simulink model "Salient_Pole_PMSG"  (R2023a)
settings: Solver=VariableStepAuto  StartTime=0.0  StopTime=10.0  RelTol=1e-3
values from neighbouring files (symbols this model uses):
  B = 0.01*Pr/(Wr^2)    (= 0.243170840742)    [SHARKS_PMSG.m]
  J = 0.2564    [SHARKS_PMSG.m]
  lamda_fd = 3*2*k/P    [SHARKS_PMSG.m]
  Lsd = 45.25e-3    (= 0.04525)    [SHARKS_PMSG.m]
  Lsq = 64.88e-3    (= 0.06488)    [SHARKS_PMSG.m]
  P = 24    [SHARKS_PMSG.m]
  Rs = 3.711    [SHARKS_PMSG.m]
libraries: spsabctodq0Lib x1
settings Model: Creator=tariq  LastModifiedBy=tariq

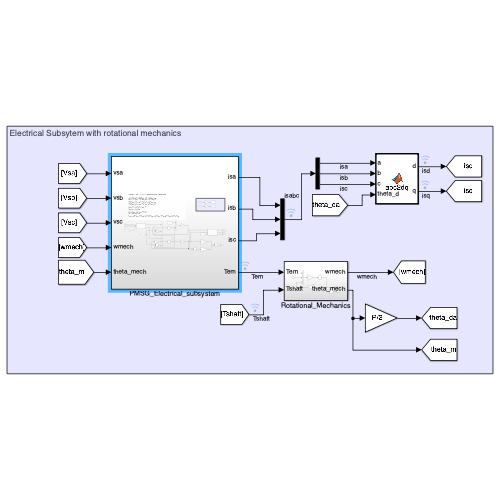
[thumbnail: Simulink's stored preview of the top-level diagram]
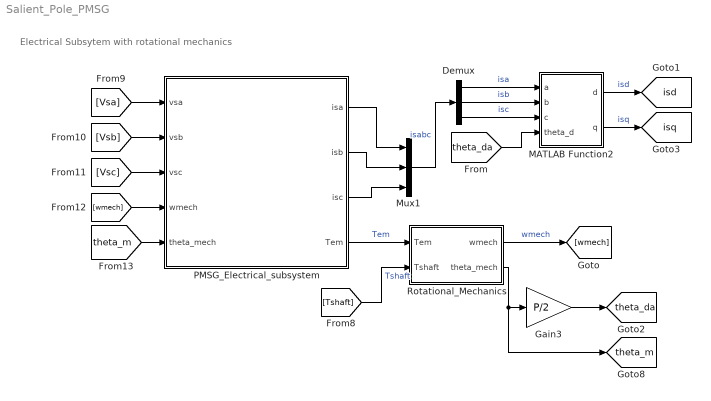
== system Salient_Pole_PMSG ==
  note: Electrical Subsytem with rotational mechanics
  Demux : Demux  Outputs=3
  Gain3 : Gain  Gain=P/2
  MATLAB Function2 : MATLAB Function  TreatAsAtomicUnit=on
  Mux1 : Mux  Inputs=3
  PMSG_Electrical_subsystem : Subsystem
  Rotational_Mechanics : Subsystem
  tag scope: isd=global, isq=global, theta_da=global, theta_m=global
  wires:
  [theta_da] -> MATLAB Function2/4(theta_d)
  Rotational_Mechanics/2(theta_mech) -> [theta_m], Gain3/1
  [Vsc] -> PMSG_Electrical_subsystem/3(vsc)
  Demux/3 -> MATLAB Function2/3(c)  "isc"
  Demux/1 -> MATLAB Function2/1(a)  "isa"
  [theta_m] -> PMSG_Electrical_subsystem/5(theta_mech)
  PMSG_Electrical_subsystem/4(Tem) -> Rotational_Mechanics/1(Tem)  "Tem"
  [Vsa] -> PMSG_Electrical_subsystem/1(vsa)
  [wmech] -> PMSG_Electrical_subsystem/4(wmech)
  MATLAB Function2/2(q) -> [isq]  "isq"
  Mux1/1 -> Demux/1  "isabc"
  [Vsb] -> PMSG_Electrical_subsystem/2(vsb)
  PMSG_Electrical_subsystem/2(isb) -> Mux1/2
  Rotational_Mechanics/1(wmech) -> [wmech]  "wmech"
  Gain3/1 -> [theta_da]
  PMSG_Electrical_subsystem/3(isc) -> Mux1/3
  MATLAB Function2/1(d) -> [isd]  "isd"
  Demux/2 -> MATLAB Function2/2(b)  "isb"
  PMSG_Electrical_subsystem/1(isa) -> Mux1/1
  [Tshaft] -> Rotational_Mechanics/2(Tshaft)  "Tshaft"

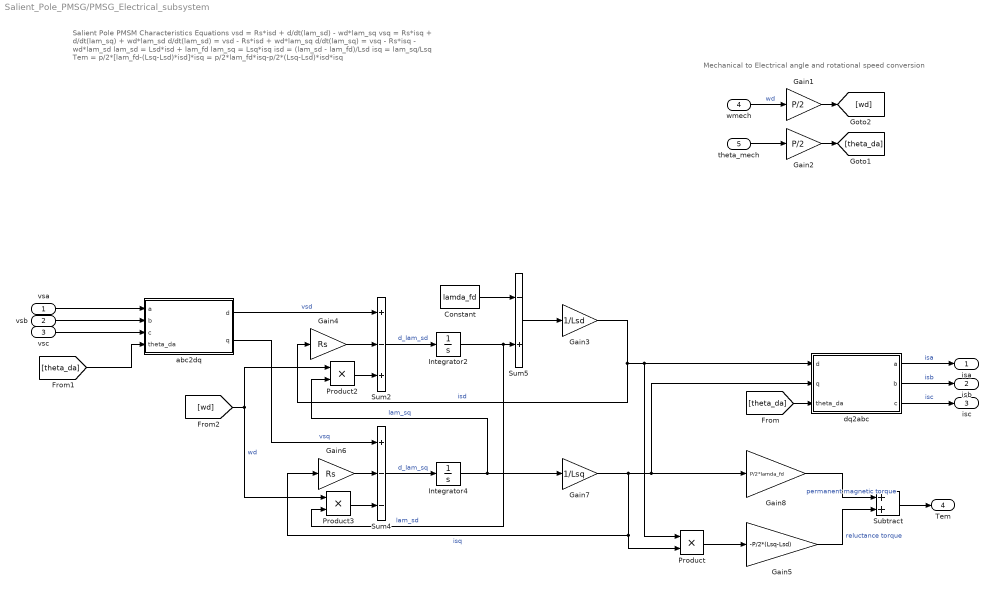
== system Salient_Pole_PMSG/PMSG_Electrical_subsystem ==
  note: Mechanical to Electrical angle and rotational speed conversion
  note: Salient Pole PMSM Characteristics Equations
      |
      | vsd = Rs*isd + d/dt(lam_sd) - wd*lam_sq
      | vsq = Rs*isq + d/dt(lam_sq) + wd*lam_sd
      |
      | d/dt(lam_sd) = vsd - Rs*isd + wd*lam_sq
      | d/dt(lam_sq) = vsq - Rs*isq - wd*lam_sd
      |
      | lam_sd = Lsd*isd + lam_fd
      | lam_sq = Lsq*isq
      |
      | isd = (lam_sd - lam_fd)/Lsd
      | isq = lam_sq/Lsq
      |
      | Tem = p/2*[lam_fd-(Lsq-Lsd)*isd]*isq = p/2*lam_fd*isq-p/2*(Lsq-Lsd)*isd*isq
  vsa : Inport
  vsb : Inport  Port=2
  vsc : Inport  Port=3
  wmech : Inport  Port=4
  theta_mech : Inport  Port=5
  Constant : Constant  Value=lamda_fd
  Gain1 : Gain  Gain=P/2
  Gain2 : Gain  Gain=P/2
  Gain3 : Gain  Gain=1/Lsd
  Gain4 : Gain  Gain=Rs
  Gain5 : Gain  Gain=-P/2*(Lsq-Lsd)
  Gain6 : Gain  Gain=Rs
  Gain7 : Gain  Gain=1/Lsq
  Gain8 : Gain  Gain=P/2*lamda_fd
  Integrator2 : Integrator
  Integrator4 : Integrator
  Product : Product
  Product2 : Product
  Product3 : Product
  Subtract : Sum
  Sum2 : Sum  Inputs=+-+
  Sum4 : Sum  Inputs=+--
  Sum5 : Sum  Inputs=-+
  abc2dq : Subsystem
  dq2abc : Subsystem
  isa : Outport  VectorParamsAs1DForOutWhenUnconnected=off
  isb : Outport  Port=2  VectorParamsAs1DForOutWhenUnconnected=off
  isc : Outport  Port=3  VectorParamsAs1DForOutWhenUnconnected=off
  Tem : Outport  Port=4  VectorParamsAs1DForOutWhenUnconnected=off
  wires:
  vsb/1 -> abc2dq/2(b)
  abc2dq/1(d) -> Sum2/1  "vsd"
  abc2dq/2(q) -> Sum4/1  "vsq"
  [theta_da] -> dq2abc/3(theta_da)
  vsc/1 -> abc2dq/3(c)
  dq2abc/1(a) -> isa/1  "isa"
  dq2abc/2(b) -> isb/1  "isb"
  Gain7/1 -> dq2abc/2(q), Gain8/1, Product/2, Gain6/1  "isq"
  dq2abc/3(c) -> isc/1  "isc"
  vsa/1 -> abc2dq/1(a)
  Gain3/1 -> Product/1, dq2abc/1(d), Gain4/1  "isd"
  Gain4/1 -> Sum2/2
  Product2/1 -> Sum2/3
  Sum2/1 -> Integrator2/1  "d_lam_sd"
  Integrator2/1 -> Product3/2, Sum5/2  "lam_sd"
  Sum4/1 -> Integrator4/1  "d_lam_sq"
  Integrator4/1 -> Product2/2, Gain7/1  "lam_sq"
  Constant/1 -> Sum5/1
  Sum5/1 -> Gain3/1
  [wd] -> Product2/1, Product3/1  "wd"
  Gain6/1 -> Sum4/2
  Product3/1 -> Sum4/3
  [theta_da] -> abc2dq/4(theta_da)
  wmech/1 -> Gain1/1  "wd"
  Gain1/1 -> [wd]
  theta_mech/1 -> Gain2/1
  Gain2/1 -> [theta_da]
  Product/1 -> Gain5/1
  Gain8/1 -> Subtract/1  "permanent magnetic torque"
  Gain5/1 -> Subtract/2  "reluctance torque"
  Subtract/1 -> Tem/1

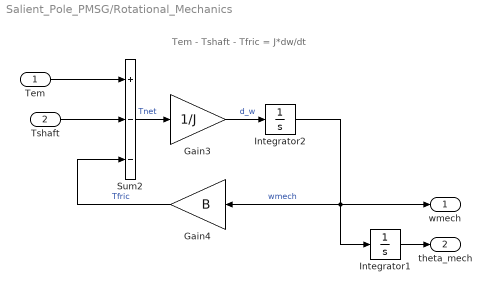
== system Salient_Pole_PMSG/Rotational_Mechanics ==
  note: Tem - Tshaft - Tfric = J*dw/dt
  Tem : Inport
  Tshaft : Inport  Port=2
  Gain3 : Gain  Gain=1/J
  Gain4 : Gain  Gain=B
  Integrator1 : Integrator  WrapState=on
  Integrator2 : Integrator
  Sum2 : Sum  Inputs=+--
  wmech : Outport  VectorParamsAs1DForOutWhenUnconnected=off
  theta_mech : Outport  Port=2  VectorParamsAs1DForOutWhenUnconnected=off
  wires:
  Tshaft/1 -> Sum2/2
  Tem/1 -> Sum2/1
  Gain4/1 -> Sum2/3  "Tfric"
  Sum2/1 -> Gain3/1  "Tnet"
  Integrator2/1 -> Integrator1/1, wmech/1, Gain4/1  "wmech"
  Gain3/1 -> Integrator2/1  "d_w"
  Integrator1/1 -> theta_mech/1

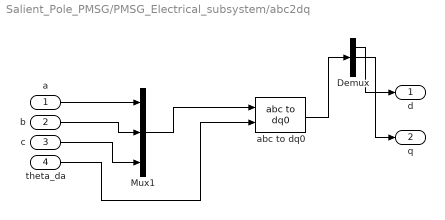
== system Salient_Pole_PMSG/PMSG_Electrical_subsystem/abc2dq ==
  a : Inport
  b : Inport  Port=2
  c : Inport  Port=3
  theta_da : Inport  Port=4
  Demux : Demux  Outputs=3
  Mux1 : Mux  Inputs=3
  abc to dq0 : spsabctodq0Lib/abc to dq0  Alignment=Aligned with phase A axis
  d : Outport  VectorParamsAs1DForOutWhenUnconnected=off
  q : Outport  Port=2  VectorParamsAs1DForOutWhenUnconnected=off
  wires:
  b/1 -> Mux1/2
  c/1 -> Mux1/3
  a/1 -> Mux1/1
  Mux1/1 -> abc to dq0/1
  theta_da/1 -> abc to dq0/2
  Demux/2 -> q/1
  Demux/1 -> d/1
  abc to dq0/1 -> Demux/1

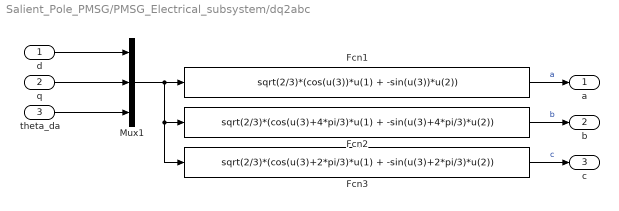
== system Salient_Pole_PMSG/PMSG_Electrical_subsystem/dq2abc ==
  d : Inport
  q : Inport  Port=2
  theta_da : Inport  Port=3
  Fcn1 : Fcn  Expr=sqrt(2/3)*(cos(u(3))*u(1) + -sin(u(3))*u(2))
  Fcn2 : Fcn  Expr=sqrt(2/3)*(cos(u(3)+4*pi/3)*u(1) + -sin(u(3)+4*pi/3)*u(2))
  Fcn3 : Fcn  Expr=sqrt(2/3)*(cos(u(3)+2*pi/3)*u(1) + -sin(u(3)+2*pi/3)*u(2))
  Mux1 : Mux  Inputs=3
  a : Outport  VectorParamsAs1DForOutWhenUnconnected=off
  b : Outport  Port=2  VectorParamsAs1DForOutWhenUnconnected=off
  c : Outport  Port=3  VectorParamsAs1DForOutWhenUnconnected=off
  wires:
  q/1 -> Mux1/2
  theta_da/1 -> Mux1/3
  Fcn2/1 -> b/1  "b"
  Fcn1/1 -> a/1  "a"
  d/1 -> Mux1/1
  Mux1/1 -> Fcn3/1, Fcn2/1, Fcn1/1
  Fcn3/1 -> c/1  "c"

== matlab function Salient_Pole_PMSG/MATLAB Function2 ==
  data: a input; d output; b input; c input; theta_d input; q output
function [d,q] = abc2dq(a,b,c,theta_d)
% Equation 12-12

d = sqrt(2/3)...
    *(...
    cos(theta_d)*a...
    + cos(theta_d - 2*pi/3)*b...
    + cos(theta_d - 4*pi/3)*c...
    ); 

q = sqrt(2/3)...
    *(...
    -sin(theta_d)*a...
    + -sin(theta_d - 2*pi/3)*b...
    + -sin(theta_d - 4*pi/3)*c...
    );
